simulink model "e01"  (R2023b)
settings: Solver=VariableStepAuto  StartTime=0.0  StopTime=10.0  RelTol=1e-3
values from neighbouring files (symbols this model uses):
  a = 1/33    (= 0.030303030303)    [e00.m]
  b = 1/33000    (= 3.0303030303e-05)    [e00.m]
  c = 0    [e00.m]
  d = 100/33    (= 3.0303030303)    [e00.m]
settings Model: Creator=jitbitan  LastModifiedBy=Anirvan Krishna

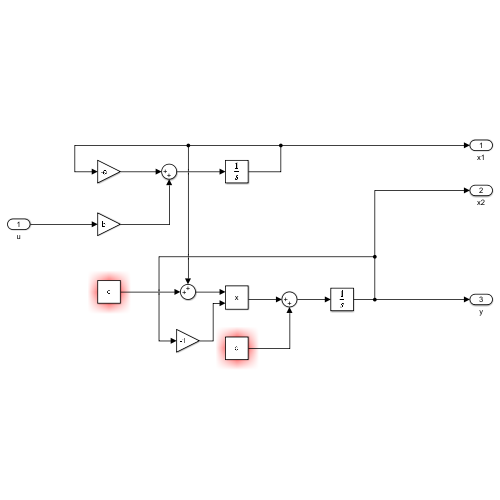
[thumbnail: Simulink's stored preview of the top-level diagram]
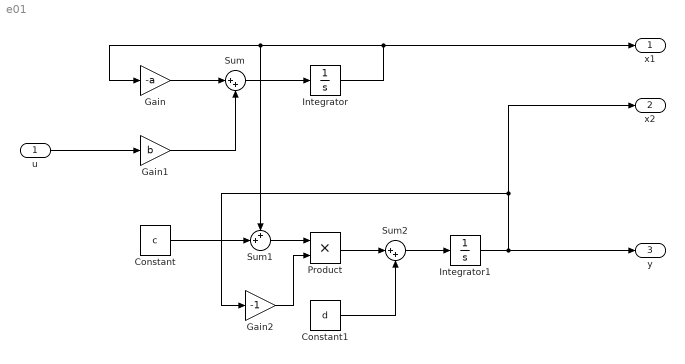
== system e01 ==
  u : Inport
  Constant : Constant  Value=c
  Constant1 : Constant  Value=d
  Gain : Gain  Gain=-a
  Gain1 : Gain  Gain=b
  Gain2 : Gain  Gain=-1
  Integrator : Integrator
  Integrator1 : Integrator
  Product : Product
  Sum : Sum  Inputs=|++
  Sum1 : Sum  Inputs=++|
  Sum2 : Sum  Inputs=|++
  x1 : Outport
  x2 : Outport  Port=2
  y : Outport  Port=3
  wires:
  Gain/1 -> Sum/1
  Gain1/1 -> Sum/2
  u/1 -> Gain1/1
  Integrator/1 -> Gain/1, Sum1/1, x1/1
  Sum/1 -> Integrator/1
  Constant/1 -> Sum1/2
  Sum1/1 -> Product/1
  Gain2/1 -> Product/2
  Integrator1/1 -> x2/1, Gain2/1, y/1
  Product/1 -> Sum2/1
  Constant1/1 -> Sum2/2
  Sum2/1 -> Integrator1/1
